simulink model "temp_control"  (R2023b)
settings: Solver=ode23t  StartTime=0.0  StopTime=t_end  RelTol=1e-3
values from neighbouring files (symbols this model uses):
  dist_gain = S.dist_gain    [mrac_control.m]    (also in run_project.m = 0.3)
  Kd = Cpid.Kd    [run_project.m]    (also in sensitivity_analysis.m = S.Kd)
  Ki = Cpid.Ki    [run_project.m]    (also in sensitivity_analysis.m = S.Ki)
  Kp = Cpid.Kp    [run_project.m]    (also in sensitivity_analysis.m = S.Kp)
  R = S.R    [mrac_control.m]    (also in run_project.m = 0.005; sensitivity_analysis.m)
  setpoint = S.setpoint    [mrac_control.m]    (also in run_project.m = 22; sensitivity_analysis.m)
  T_amb = S.T_amb    [mrac_control.m]    (also in run_project.m = 5; sensitivity_analysis.m)
  tau = S.tau    [mrac_control.m]    (also in run_project.m = 600; sensitivity_analysis.m)
  tau2 = S.tau2    [mrac_control.m]    (also in run_project.m = 30; sensitivity_analysis.m)
  u_max = S.u_max    [mrac_control.m]    (also in run_project.m = 8000; sensitivity_analysis.m)
libraries: slpidlib x1
settings Model: Creator=Korisnik  LastModifiedBy=Korisnik

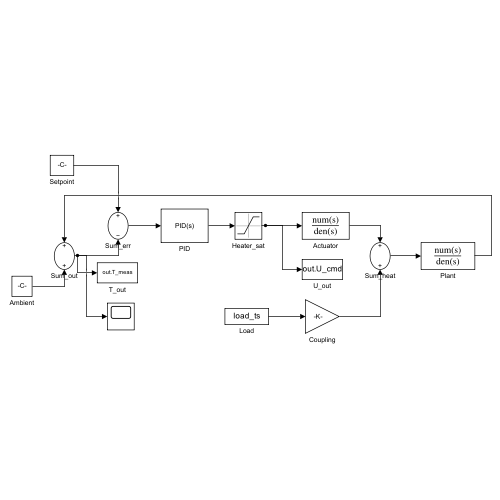
[thumbnail: Simulink's stored preview of the top-level diagram]
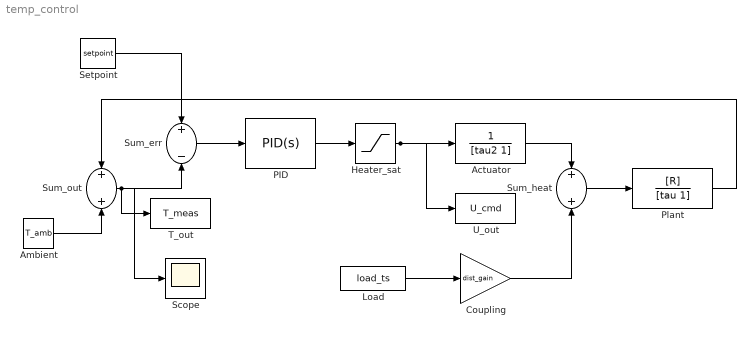
== system temp_control ==
  Actuator : TransferFcn  Denominator=[tau2 1]
  Ambient : Constant  Value=T_amb
  Coupling : Gain  Gain=dist_gain
  Heater_sat : Saturate  UpperLimit=u_max  LowerLimit=0
  Load : FromWorkspace  VariableName=load_ts  OutputAfterFinalValue=Holding final value
  PID : slpidlib/PID Controller  Controller=PID  Form=Parallel  TimeDomain=Continuous-time  UseExternalTs=off  SampleTime=-1  IntegratorMethod=Forward Euler  FilterMethod=Forward Euler  ControllerParametersSource=internal  P=Kp  I=Ki  UseKiTs=off  D=Kd  N=100  UseFilter=on  TunerSelectOption=Transfer Function Based (PID Tuner App)  InitialConditionSource=internal  InitialConditionForIntegrator=0  InitialConditionForFilter=0  DifferentiatorICPrevScaledInput=0  ExternalReset=none  TrackingMode=off  Kt=1  LimitOutput=off  SatLimitsSource=internal  UpperSaturationLimit=inf  LowerSaturationLimit=-inf  LinearizeAsGain=on  AntiWindupMode=none  Kb=1  LimitIntegrator=off  UpperIntegratorSaturationLimit=inf  LowerIntegratorSaturationLimit=-inf  POutMin=[]  POutMax=[]  IOutMin=[]  IOutMax=[]  DOutMin=[]  DOutMax=[]  NOutMin=[]  NOutMax=[]  SumOutMin=[]  SumOutMax=[]  SaturationOutMin=[]  SaturationOutMax=[]  PParamMin=[]  PParamMax=[]  IParamMin=[]  IParamMax=[]  DParamMin=[]  DParamMax=[]  NParamMin=[]  NParamMax=[]  KbParamMin=[]  KbParamMax=[]  KtParamMin=[]  KtParamMax=[]  KbOutMin=[]  KbOutMax=[]  KtOutMin=[]  KtOutMax=[]  IntegratorOutMin=[]  IntegratorOutMax=[]  FilterOutMin=[]  FilterOutMax=[]  SumI1OutMin=[]  SumI1OutMax=[]  SumI2OutMin=[]  SumI2OutMax=[]  SumI3OutMin=[]  SumI3OutMax=[]  SumI4OutMin=[]  SumI4OutMax=[]  SumDOutMin=[]  SumDOutMax=[]  DifferentiatorOutMin=[]  DifferentiatorOutMax=[]  FilterDiffOutCoefMin=[]  FilterDiffOutCoefMax=[]  ReciprocalOutMin=[]  ReciprocalOutMax=[]  SumDenOutMin=[]  SumDenOutMax=[]  SumNumOutMin=[]  SumNumOutMax=[]  DivideOutMin=[]  DivideOutMax=[]  UdiffTsProdOutMin=[]  UdiffTsProdOutMax=[]  NTsProdOutMin=[]  NTsProdOutMax=[]  UintegralTsProdOutMin=[]  UintegralTsProdOutMax=[]  UngainTsProdOutMin=[]  UngainTsProdOutMax=[]  ClampingZeroOutDataTypeStr=Inherit: Inherit via back propagation  ClampingZeroOutMin=[]  ClampingZeroOutMax=[]  FilterDenConstantOutDataTypeStr=Inherit: Inherit via back propagation  FilterDenConstantOutMin=[]  FilterDenConstantOutMax=[]  PCopyOutDataTypeStr=Inherit: Inherit via back propagation  PCopyOutMin=[]  PCopyOutMax=[]  NCopyOutDataTypeStr=Inherit: Inherit via back propagation  NCopyOutMin=[]  NCopyOutMax=[]  IntegratorContinuousStateAttributes=''  IntegratorStateMustResolveToSignalObject=off  IntegratorRTWStateStorageClass=Auto  FilterContinuousStateAttributes=''  FilterStateMustResolveToSignalObject=off  FilterRTWStateStorageClass=Auto  ParallelPVariant=InternalParameters  IdealPVariant=Disabled  IVariant=InternalParameters  DVariant=InternalParameters  IntegratorVariant=Continuous  SatVariant=Disabled  AWVariant=Passthrough  PCopyVariant=Disabled  TRVariant=Disabled  FdbkBlocksVariant=Forward  IdealPFdbkVariant=Disabled  SatFdbkVariant=Disabled  DerivativeFilterVariant=ContFilter  NVariant=InternalParameters  NCopyVariant=Disabled  FilterICVariant=InternalICsFilter  IntegratorICVariant=InternalICs  ExternalResetVariant=Disabled  TRSumVariant=Passthrough  SumFdbkVariant=Disabled  SumVariant=Sum_PID  TsampFilterVariant=InternalTs  TsampNgainVariant=Passthrough  TsampIntegralVariant=Disabled_SignalSpec  ExternalSaturationOutDataTypeStr=Inherit: Same as second input
  Plant : TransferFcn  Numerator=[R]  Denominator=[tau 1]
  Scope : Scope
  Setpoint : Constant  Value=setpoint
  Sum_err : Sum  Inputs=+-
  Sum_heat : Sum
  Sum_out : Sum
  T_out : ToWorkspace  VariableName=T_meas  SaveFormat=Timeseries  SampleTime=-1
  U_out : ToWorkspace  VariableName=U_cmd  SaveFormat=Timeseries  SampleTime=-1
  wires:
  Heater_sat/1 -> U_out/1, Actuator/1
  Sum_out/1 -> Sum_err/2, Scope/1, T_out/1
  Ambient/1 -> Sum_out/2
  Actuator/1 -> Sum_heat/1
  PID/1 -> Heater_sat/1
  Setpoint/1 -> Sum_err/1
  Sum_err/1 -> PID/1
  Load/1 -> Coupling/1
  Coupling/1 -> Sum_heat/2
  Sum_heat/1 -> Plant/1
  Plant/1 -> Sum_out/1
